simulink model "dual_mode_avg_TB"  (R2024a)
settings: Solver=VariableStepAuto  StartTime=0.0  StopTime=2000  RelTol=1e-3
PreLoadFcn:
  | N = 100;
InitFcn:
  | N = 100;
libraries: simulink x1, dspsrcs4 x1
settings Model: Creator=kschutz  LastModifiedBy=kschutz

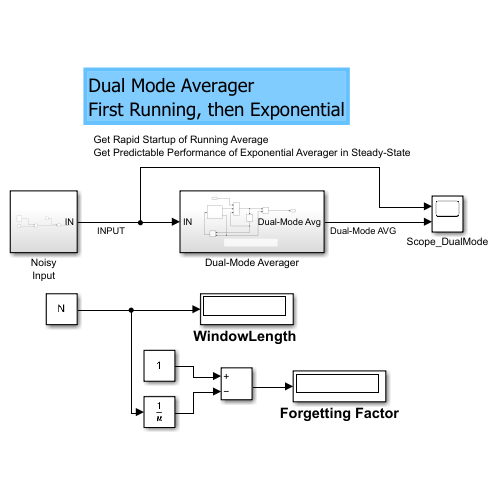
[thumbnail: Simulink's stored preview of the top-level diagram]
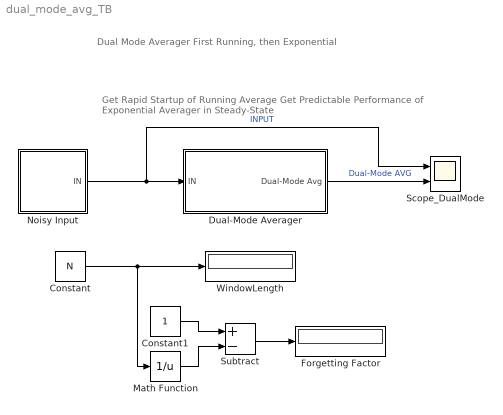
== system dual_mode_avg_TB ==
  note: Dual Mode Averager
      | First Running, then Exponential
  note: Get Rapid Startup of Running Average
      | Get Predictable Performance of Exponential Averager in Steady-State
  Constant : Constant  Value=N
  Constant1 : Constant
  Dual-Mode Averager : Subsystem
  Forgetting Factor : Display
  Math Function : Math  Operator=reciprocal
  Noisy Input : Subsystem
  Scope_DualMode : Scope  NumInputPorts=2
  Subtract : Sum  Inputs=+-
  "WindowLength " : Display
  wires:
  Dual-Mode Averager/1(Dual-Mode Avg) -> Scope_DualMode/2  "Dual-Mode AVG"
  Noisy Input/1(IN) -> Scope_DualMode/1, Dual-Mode Averager/1(IN)  "INPUT"
  Constant/1 -> "WindowLength "/1, Math Function/1
  Math Function/1 -> Subtract/2
  Constant1/1 -> Subtract/1
  Subtract/1 -> Forgetting Factor/1

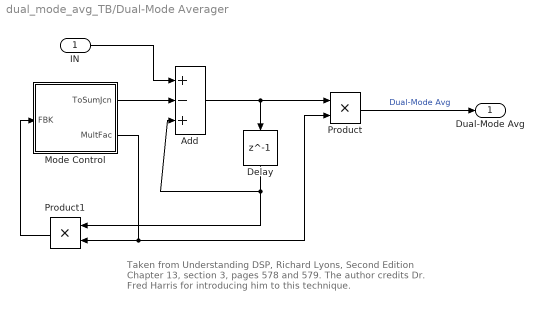
== system dual_mode_avg_TB/Dual-Mode Averager ==
  note: Taken from Understanding DSP, Richard Lyons, Second Edition
      | Chapter 13, section 3, pages 578 and 579. The author credits
      | Dr. Fred Harris for introducing him to this technique.
  IN : Inport
  Add : Sum  Inputs=+-+
  Delay : Delay  DelayLength=1
  Mode Control : Subsystem
  Product : Product
  Product1 : Product
  Dual-Mode Avg : Outport  VectorParamsAs1DForOutWhenUnconnected=off
  wires:
  Add/1 -> Product/1, Delay/1
  Mode Control/2(MultFac) -> Product1/2, Product/2
  Delay/1 -> Product1/1, Add/3
  Mode Control/1(ToSumJcn) -> Add/2
  Product/1 -> Dual-Mode Avg/1  "Dual-Mode Avg"
  IN/1 -> Add/1
  Product1/1 -> Mode Control/1(FBK)

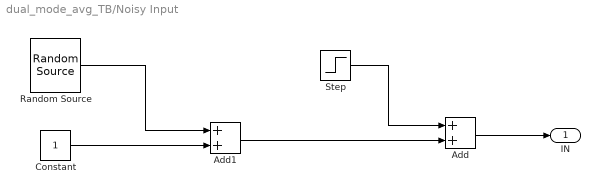
== system dual_mode_avg_TB/Noisy Input ==
  Add : Sum
  Add1 : Sum
  Constant : Constant  SampleTime=1
  Random Source : dspsrcs4/Random Source  SrcType=Gaussian  MinVal=0  MaxVal=1  MeanVal=0  VarVal=.2  RepMode=Specify seed  rawSeed=123  IsInherit=off  SampTime=1  SampFrame=1  OutComplex=Real  DataType=double  SimulateUsing=Interpreted execution
  Step : Step  Time=500  SampleTime=0
  IN : Outport  VectorParamsAs1DForOutWhenUnconnected=off
  wires:
  Constant/1 -> Add1/2
  Random Source/1 -> Add1/1
  Add/1 -> IN/1
  Add1/1 -> Add/2
  Step/1 -> Add/1

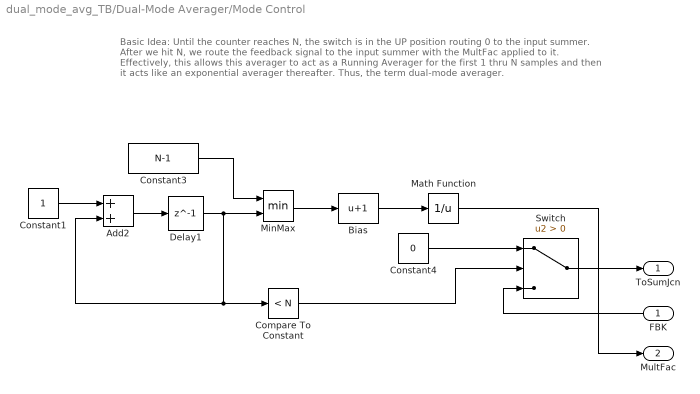
== system dual_mode_avg_TB/Dual-Mode Averager/Mode Control ==
  note: Basic Idea: Until the counter reaches N, the switch is in the UP position routing 0 to the input summer.
      | After we hit N, we route the feedback signal to the input summer with the MultFac applied to it.
      | Effectively, this allows this averager to act as a Running Averager for the first 1 thru N samples
      | and then it acts like an exponential averager thereafter. Thus, the term dual-mode averager.
  FBK : Inport
  Add2 : Sum
  Bias : Bias  Bias=1  SaturateOnIntegerOverflow=off
  Compare To Constant : simulink/Logic and Bit Operations/Compare To Constant  relop=<  const=N  OutDataTypeStr=boolean
  Constant1 : Constant
  Constant3 : Constant  Value=N-1  OutDataTypeStr=single  SampleTime=1
  Constant4 : Constant  Value=0
  Delay1 : Delay  DelayLength=1  InitialCondition=0
  Math Function : Math  Operator=reciprocal  SignedPower=on
  MinMax : MinMax  Inputs=2
  Switch : Switch  Criteria=u2 > Threshold  SaturateOnIntegerOverflow=off  InputSameDT=off
  ToSumJcn : Outport  VectorParamsAs1DForOutWhenUnconnected=off
  MultFac : Outport  Port=2  VectorParamsAs1DForOutWhenUnconnected=off
  wires:
  Delay1/1 -> MinMax/2, Compare To Constant/1, Add2/2
  Switch/1 -> ToSumJcn/1
  Add2/1 -> Delay1/1
  Constant1/1 -> Add2/1
  Bias/1 -> Math Function/1
  MinMax/1 -> Bias/1
  Constant4/1 -> Switch/1
  Constant3/1 -> MinMax/1
  Compare To Constant/1 -> Switch/2
  FBK/1 -> Switch/3
  Math Function/1 -> MultFac/1
